simulink model "DC_motor_MPC"  (R2023a)
settings: Solver=FixedStepAuto  StartTime=0.0  StopTime=inf  FixedStep=0.002  RelTol=1e-3  EnableMultiTasking=on
values from neighbouring files (symbols this model uses):
  Npred = 20    [MPC_CasADi_2.m]
  Ts = 0.02    [MPC_CasADi_2.m]
undefined symbols (not defined in the file or in its folder): HIL, qc_get_step_size
libraries: quarc_library x33, dspbuff3 x12, simulink x7
settings Model: Creator=bajdus  LastModifiedBy=marinst
settings SolverCC: PositivePriorityOrder=on  AutoInsertRateTranBlk=on
settings RTWCC: Description=QUARC Win64 Target Using Toolchain  SystemTargetFile=quarc_win64.tlc  Toolchain=QUARC win64 | nmake (64-bit Windows)  BuildConfiguration=Faster Runs
settings STFCustomTargetCC: SystemTargetFile=quarc_win64.tlc
settings GRTTargetCC: ParMdlRefBuildCompliant=off  CompOptLevelCompliant=off  CombineOutputUpdateFcns=off  MatFileLogging=off  CPPClassGenCompliant=off  GRTInterface=on  ExtMode=on  ExtModeMexFile=quarc_comm

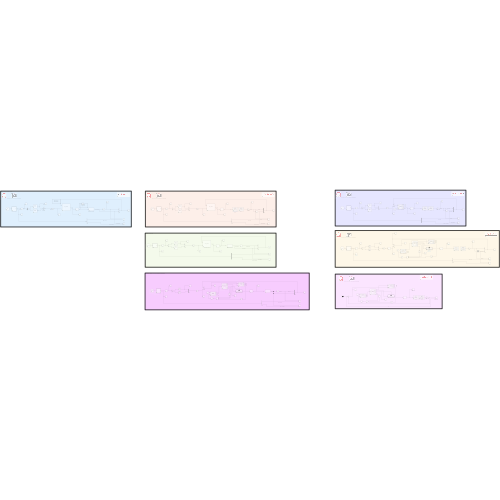
[thumbnail: Simulink's stored preview of the top-level diagram]
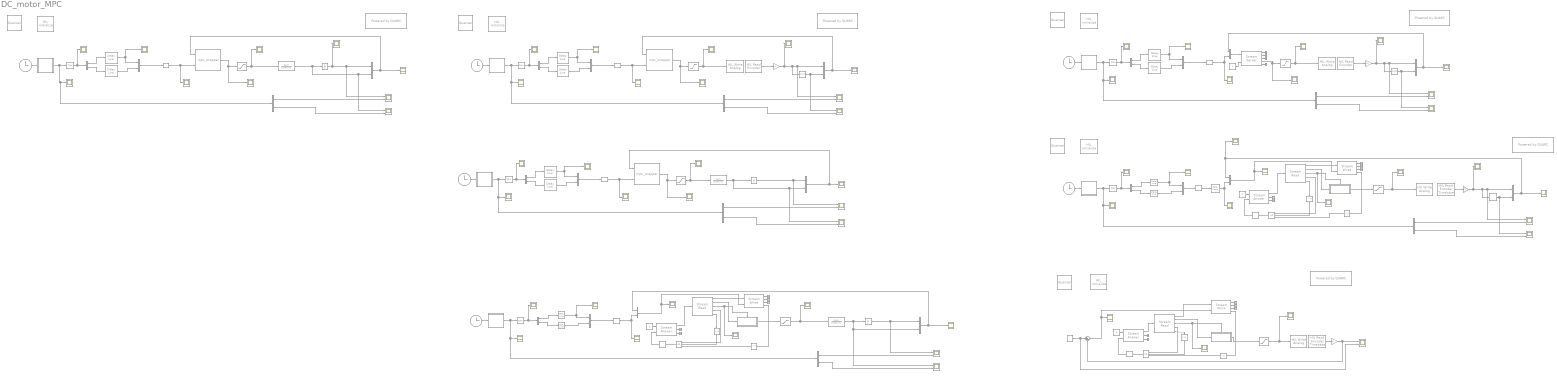
== system DC_motor_MPC ==
  note: QUARC Model PID - Server. Intermediate Communication
  note: Transfer function model
  note: QUARC Model
  note: QUARC Mode - Server. Basic Communication
  note: QUARC Model - Server. Intermediate Communication
  note: Mathematical Model - Server. Intermediate Communication
  note: QUARC Model - Transfer Function
  CasADi S-Function : S-Function  Commented=on  FunctionName=mpc_wrapper  SFunctionDeploymentMode=off  EnableBusSupport=off
  CasADi S-Function1 : S-Function  Commented=on  FunctionName=mpc_wrapper  SFunctionDeploymentMode=off  EnableBusSupport=off
  CasADi S-Function2 : S-Function  Commented=on  FunctionName=mpc_wrapper  SFunctionDeploymentMode=off  EnableBusSupport=off
  Clock{,1..5} (6 alike) : Clock  Commented=on
  Compare To Zero{,1..5} (6 alike) : simulink/Logic and Bit Operations/Compare To Zero  Commented=on  relop=<  OutDataTypeStr=boolean
  Constant : Constant  Commented=on
  Constant1 : Constant  Commented=on  Value=0
  Constant2 : Constant  Commented=on  Value=0
  Constant3 : Constant  Commented=on  Value=0
  Delay Line{,1..11} (12 alike) : dspbuff3/Delay Line  Commented=on  siz=Npred+1  ic=0  directfeed=off  enable_output=off  hold_output=off  OutputFrames=off
  Demux{,1..11} (12 alike) : Demux  Commented=on  Outputs=2
  Derivative : Derivative  Commented=on
  Derivative1 : Derivative  Commented=on
  Discrete Derivative : simulink/Discrete/Discrete Derivative  Commented=on  gainval=1.0  ICPrevScaledInput=0.0  OutMin=[]  OutMax=[]  OutDataType=fixdt(1, 16)  OutScaling=2^-10  DoSatur=off
  Enabled Subsystem : Subsystem  Commented=on  TreatAsAtomicUnit=on
  Enabled Subsystem1 : Subsystem  Commented=on  TreatAsAtomicUnit=on
  Enabled Subsystem2 : Subsystem  Commented=on  TreatAsAtomicUnit=on
  HIL Initialize : quarc_library/Data Acquisition/Generic/Configuration/HIL Initialize  Priority=-99  Commented=on  object_name=HIL-1  board_type=qube_servo3_usb  board_number=0@tcpip://localhost:18922  board_options=deadband_compensation=0.3;pwm_en=0;enc0_velocity=3.0;enc1_velocity=3.0;min_diode_compensation=0.3;max_diode_compensation=1.5  exclusive=off  active=off  hardware_clocks=[0]  clock_modes=[]  initial_clock_frequencies=[]  set_clock_params_at_start=off  set_clock_params_at_switch_in=off  set_clock_frequencies_at_start=off  set_clock_frequencies_at_switch_in=off  analog_input_channels=[0]  analog_input_configurations=[]  analog_input_maximums=3  analog_input_minimums=-3  set_analog_input_params_at_start=off  set_analog_input_params_at_switch_in=off  analog_output_channels=[0]  analog_output_maximums=15  analog_output_minimums=-15  initial_analog_outputs=[0]  final_analog_outputs=[0]  watchdog_analog_outputs=0  set_analog_output_params_at_start=off  set_analog_output_params_at_switch_in=off  set_analog_outputs_at_start=on  set_analog_outputs_at_switch_in=off  set_analog_outputs_at_terminate=on  set_analog_outputs_at_switch_out=off  set_analog_outputs_on_watchdog=on  digital_input_channels=[]  digital_output_channels=[0]  digital_output_configuration=[]  initial_digital_outputs=[1]  final_digital_outputs=[0]  watchdog_digital_outputs=[0]  set_digital_output_params_at_start=off  set_digital_output_params_at_switch_in=off  set_digital_outputs_at_start=on  set_digital_outputs_at_switch_in=off  set_digital_outputs_at_terminate=on  set_digital_outputs_at_switch_out=off  set_digital_outputs_on_watchdog=on  encoder_channels=[0:1]  quadrature=[4]  encoder_filter_frequency=[]  initial_encoder_counts=[0]  set_encoder_params_at_start=off  set_encoder_params_at_switch_in=off  set_encoder_counts_at_start=on  set_encoder_counts_at_switch_in=off  pwm_channels=[]  pwm_modes=[0]  pwm_frequency=23195  pwm_configuration=[1]  pwm_alignment=[0]  pwm_polarity=[1]  pwm_leading_deadband=[0]  pwm_trailing_deadband=[0]  initial_pwm_outputs=[0]  final_pwm_outputs=[0]  watchdog_pwm_outputs=[]  set_pwm_params_at_start=off  set_pwm_params_at_switch_in=off  set_pwm_outputs_at_start=off  set_pwm_outputs_at_switch_in=off  set_pwm_outputs_at_terminate=off  set_pwm_outputs_at_switch_out=off  set_pwm_outputs_on_watchdog=off  other_output_channels=[11000:11002]  initial_other_outputs=[0 1 0]  final_other_outputs=[1 0 0]  watchdog_other_outputs=[0 0 1]  set_other_outputs_at_start=on  set_other_outputs_at_switch_in=off  set_other_outputs_at_terminate=on  set_other_outputs_at_switch_out=off  set_other_outputs_on_watchdog=on
  HIL Initialize1 : quarc_library/Data Acquisition/Generic/Configuration/HIL Initialize  Priority=-99  Commented=on  object_name=HIL-1  board_type=qube_servo3_usb  board_number=0@tcpip://localhost:18922  board_options=deadband_compensation=0.3;pwm_en=0;enc0_velocity=3.0;enc1_velocity=3.0;min_diode_compensation=0.3;max_diode_compensation=1.5  exclusive=off  active=off  hardware_clocks=[0]  clock_modes=[]  initial_clock_frequencies=[]  set_clock_params_at_start=off  set_clock_params_at_switch_in=off  set_clock_frequencies_at_start=off  set_clock_frequencies_at_switch_in=off  analog_input_channels=[0]  analog_input_configurations=[]  analog_input_maximums=3  analog_input_minimums=-3  set_analog_input_params_at_start=off  set_analog_input_params_at_switch_in=off  analog_output_channels=[0]  analog_output_maximums=15  analog_output_minimums=-15  initial_analog_outputs=[0]  final_analog_outputs=[0]  watchdog_analog_outputs=0  set_analog_output_params_at_start=off  set_analog_output_params_at_switch_in=off  set_analog_outputs_at_start=on  set_analog_outputs_at_switch_in=off  set_analog_outputs_at_terminate=on  set_analog_outputs_at_switch_out=off  set_analog_outputs_on_watchdog=on  digital_input_channels=[]  digital_output_channels=[0]  digital_output_configuration=[]  initial_digital_outputs=[1]  final_digital_outputs=[0]  watchdog_digital_outputs=[0]  set_digital_output_params_at_start=off  set_digital_output_params_at_switch_in=off  set_digital_outputs_at_start=on  set_digital_outputs_at_switch_in=off  set_digital_outputs_at_terminate=on  set_digital_outputs_at_switch_out=off  set_digital_outputs_on_watchdog=on  encoder_channels=[0:1]  quadrature=[4]  encoder_filter_frequency=[]  initial_encoder_counts=[0]  set_encoder_params_at_start=off  set_encoder_params_at_switch_in=off  set_encoder_counts_at_start=on  set_encoder_counts_at_switch_in=off  pwm_channels=[]  pwm_modes=[0]  pwm_frequency=23195  pwm_configuration=[1]  pwm_alignment=[0]  pwm_polarity=[1]  pwm_leading_deadband=[0]  pwm_trailing_deadband=[0]  initial_pwm_outputs=[0]  final_pwm_outputs=[0]  watchdog_pwm_outputs=[]  set_pwm_params_at_start=off  set_pwm_params_at_switch_in=off  set_pwm_outputs_at_start=off  set_pwm_outputs_at_switch_in=off  set_pwm_outputs_at_terminate=off  set_pwm_outputs_at_switch_out=off  set_pwm_outputs_on_watchdog=off  other_output_channels=[11000:11002]  initial_other_outputs=[0 1 0]  final_other_outputs=[1 0 0]  watchdog_other_outputs=[0 0 1]  set_other_outputs_at_start=on  set_other_outputs_at_switch_in=off  set_other_outputs_at_terminate=on  set_other_outputs_at_switch_out=off  set_other_outputs_on_watchdog=on
  HIL Initialize2 : quarc_library/Data Acquisition/Generic/Configuration/HIL Initialize  Priority=-99  Commented=on  object_name=HIL-2  board_type=qube_servo3_usb  board_number=0@tcpip://localhost:18922  board_options=deadband_compensation=0.3;pwm_en=0;enc0_velocity=3.0;enc1_velocity=3.0;min_diode_compensation=0.3;max_diode_compensation=1.5  exclusive=off  active=off  hardware_clocks=[0]  clock_modes=[]  initial_clock_frequencies=[]  set_clock_params_at_start=off  set_clock_params_at_switch_in=off  set_clock_frequencies_at_start=off  set_clock_frequencies_at_switch_in=off  analog_input_channels=[0]  analog_input_configurations=[]  analog_input_maximums=3  analog_input_minimums=-3  set_analog_input_params_at_start=off  set_analog_input_params_at_switch_in=off  analog_output_channels=[0]  analog_output_maximums=15  analog_output_minimums=-15  initial_analog_outputs=[0]  final_analog_outputs=[0]  watchdog_analog_outputs=0  set_analog_output_params_at_start=off  set_analog_output_params_at_switch_in=off  set_analog_outputs_at_start=on  set_analog_outputs_at_switch_in=off  set_analog_outputs_at_terminate=on  set_analog_outputs_at_switch_out=off  set_analog_outputs_on_watchdog=on  digital_input_channels=[]  digital_output_channels=[0]  digital_output_configuration=[]  initial_digital_outputs=[1]  final_digital_outputs=[0]  watchdog_digital_outputs=[0]  set_digital_output_params_at_start=off  set_digital_output_params_at_switch_in=off  set_digital_outputs_at_start=on  set_digital_outputs_at_switch_in=off  set_digital_outputs_at_terminate=on  set_digital_outputs_at_switch_out=off  set_digital_outputs_on_watchdog=on  encoder_channels=[0:1]  quadrature=[4]  encoder_filter_frequency=[]  initial_encoder_counts=[0]  set_encoder_params_at_start=off  set_encoder_params_at_switch_in=off  set_encoder_counts_at_start=on  set_encoder_counts_at_switch_in=off  pwm_channels=[]  pwm_modes=[0]  pwm_frequency=23195  pwm_configuration=[1]  pwm_alignment=[0]  pwm_polarity=[1]  pwm_leading_deadband=[0]  pwm_trailing_deadband=[0]  initial_pwm_outputs=[0]  final_pwm_outputs=[0]  watchdog_pwm_outputs=[]  set_pwm_params_at_start=off  set_pwm_params_at_switch_in=off  set_pwm_outputs_at_start=off  set_pwm_outputs_at_switch_in=off  set_pwm_outputs_at_terminate=off  set_pwm_outputs_at_switch_out=off  set_pwm_outputs_on_watchdog=off  other_output_channels=[11000:11002]  initial_other_outputs=[0 1 0]  final_other_outputs=[1 0 0]  watchdog_other_outputs=[0 0 1]  set_other_outputs_at_start=on  set_other_outputs_at_switch_in=off  set_other_outputs_at_terminate=on  set_other_outputs_at_switch_out=off  set_other_outputs_on_watchdog=on
  HIL Initialize3 : quarc_library/Data Acquisition/Generic/Configuration/HIL Initialize  Priority=-99  Commented=on  object_name=HIL-1  board_type=qube_servo3_usb  board_number=0@tcpip://localhost:18922  board_options=deadband_compensation=0.3;pwm_en=0;enc0_velocity=3.0;enc1_velocity=3.0;min_diode_compensation=0.3;max_diode_compensation=1.5  exclusive=off  active=off  hardware_clocks=[0]  clock_modes=[]  initial_clock_frequencies=[]  set_clock_params_at_start=off  set_clock_params_at_switch_in=off  set_clock_frequencies_at_start=off  set_clock_frequencies_at_switch_in=off  analog_input_channels=[0]  analog_input_configurations=[]  analog_input_maximums=3  analog_input_minimums=-3  set_analog_input_params_at_start=off  set_analog_input_params_at_switch_in=off  analog_output_channels=[0]  analog_output_maximums=15  analog_output_minimums=-15  initial_analog_outputs=[0]  final_analog_outputs=[0]  watchdog_analog_outputs=0  set_analog_output_params_at_start=off  set_analog_output_params_at_switch_in=off  set_analog_outputs_at_start=on  set_analog_outputs_at_switch_in=off  set_analog_outputs_at_terminate=on  set_analog_outputs_at_switch_out=off  set_analog_outputs_on_watchdog=on  digital_input_channels=[]  digital_output_channels=[0]  digital_output_configuration=[]  initial_digital_outputs=[1]  final_digital_outputs=[0]  watchdog_digital_outputs=[0]  set_digital_output_params_at_start=off  set_digital_output_params_at_switch_in=off  set_digital_outputs_at_start=on  set_digital_outputs_at_switch_in=off  set_digital_outputs_at_terminate=on  set_digital_outputs_at_switch_out=off  set_digital_outputs_on_watchdog=on  encoder_channels=[0:1]  quadrature=[4]  encoder_filter_frequency=[]  initial_encoder_counts=[0]  set_encoder_params_at_start=off  set_encoder_params_at_switch_in=off  set_encoder_counts_at_start=on  set_encoder_counts_at_switch_in=off  pwm_channels=[]  pwm_modes=[0]  pwm_frequency=23195  pwm_configuration=[1]  pwm_alignment=[0]  pwm_polarity=[1]  pwm_leading_deadband=[0]  pwm_trailing_deadband=[0]  initial_pwm_outputs=[0]  final_pwm_outputs=[0]  watchdog_pwm_outputs=[]  set_pwm_params_at_start=off  set_pwm_params_at_switch_in=off  set_pwm_outputs_at_start=off  set_pwm_outputs_at_switch_in=off  set_pwm_outputs_at_terminate=off  set_pwm_outputs_at_switch_out=off  set_pwm_outputs_on_watchdog=off  other_output_channels=[11000:11002]  initial_other_outputs=[0 1 0]  final_other_outputs=[1 0 0]  watchdog_other_outputs=[0 0 1]  set_other_outputs_at_start=on  set_other_outputs_at_switch_in=off  set_other_outputs_at_terminate=on  set_other_outputs_at_switch_out=off  set_other_outputs_on_watchdog=on
  HIL Initialize4 : quarc_library/Data Acquisition/Generic/Configuration/HIL Initialize  Priority=-99  Commented=on  object_name=HIL-2  board_type=qube_servo3_usb  board_number=0@tcpip://localhost:18922  board_options=deadband_compensation=0.3;pwm_en=0;enc0_velocity=3.0;enc1_velocity=3.0;min_diode_compensation=0.3;max_diode_compensation=1.5  exclusive=off  active=off  hardware_clocks=[0]  clock_modes=[]  initial_clock_frequencies=[]  set_clock_params_at_start=off  set_clock_params_at_switch_in=off  set_clock_frequencies_at_start=off  set_clock_frequencies_at_switch_in=off  analog_input_channels=[0]  analog_input_configurations=[]  analog_input_maximums=3  analog_input_minimums=-3  set_analog_input_params_at_start=off  set_analog_input_params_at_switch_in=off  analog_output_channels=[0]  analog_output_maximums=15  analog_output_minimums=-15  initial_analog_outputs=[0]  final_analog_outputs=[0]  watchdog_analog_outputs=0  set_analog_output_params_at_start=off  set_analog_output_params_at_switch_in=off  set_analog_outputs_at_start=on  set_analog_outputs_at_switch_in=off  set_analog_outputs_at_terminate=on  set_analog_outputs_at_switch_out=off  set_analog_outputs_on_watchdog=on  digital_input_channels=[]  digital_output_channels=[0]  digital_output_configuration=[]  initial_digital_outputs=[1]  final_digital_outputs=[0]  watchdog_digital_outputs=[0]  set_digital_output_params_at_start=off  set_digital_output_params_at_switch_in=off  set_digital_outputs_at_start=on  set_digital_outputs_at_switch_in=off  set_digital_outputs_at_terminate=on  set_digital_outputs_at_switch_out=off  set_digital_outputs_on_watchdog=on  encoder_channels=[0:1]  quadrature=[4]  encoder_filter_frequency=[]  initial_encoder_counts=[0]  set_encoder_params_at_start=off  set_encoder_params_at_switch_in=off  set_encoder_counts_at_start=on  set_encoder_counts_at_switch_in=off  pwm_channels=[]  pwm_modes=[0]  pwm_frequency=23195  pwm_configuration=[1]  pwm_alignment=[0]  pwm_polarity=[1]  pwm_leading_deadband=[0]  pwm_trailing_deadband=[0]  initial_pwm_outputs=[0]  final_pwm_outputs=[0]  watchdog_pwm_outputs=[]  set_pwm_params_at_start=off  set_pwm_params_at_switch_in=off  set_pwm_outputs_at_start=off  set_pwm_outputs_at_switch_in=off  set_pwm_outputs_at_terminate=off  set_pwm_outputs_at_switch_out=off  set_pwm_outputs_on_watchdog=off  other_output_channels=[11000:11002]  initial_other_outputs=[0 1 0]  final_other_outputs=[1 0 0]  watchdog_other_outputs=[0 0 1]  set_other_outputs_at_start=on  set_other_outputs_at_switch_in=off  set_other_outputs_at_terminate=on  set_other_outputs_at_switch_out=off  set_other_outputs_on_watchdog=on
  HIL Read Encoder : quarc_library/Data Acquisition/Generic/Immediate I//O/HIL Read Encoder  Commented=on  object_name=HIL-1  channels=0  sample_time=qc_get_step_size  active=on  vector_output=off  data_type_mode=Inherit via back propagation  data_type=double
  HIL Read Encoder Timebase : quarc_library/Data Acquisition/Generic/Timebases/HIL Read Encoder Timebase  Commented=on  object_name=HIL-2  clock=0  channels=0  active=on  vector_output=off  data_type_mode=Inherit via back propagation  data_type=double  overflow_mode=Error on overflow  samples_in_buffer=max(ceil(1/qc_get_step_size), 1)
  HIL Read Encoder Timebase1 : quarc_library/Data Acquisition/Generic/Timebases/HIL Read Encoder Timebase  Commented=on  object_name=HIL-1  clock=0  channels=0  active=on  vector_output=off  data_type_mode=Inherit via back propagation  data_type=double  overflow_mode=Error on overflow  samples_in_buffer=max(ceil(1/qc_get_step_size), 1)
  HIL Read Encoder1 : quarc_library/Data Acquisition/Generic/Immediate I//O/HIL Read Encoder  Commented=on  object_name=HIL-1  channels=0  sample_time=qc_get_step_size  active=on  vector_output=off  data_type_mode=Inherit via back propagation  data_type=double
  HIL Write Analog : quarc_library/Data Acquisition/Generic/Immediate I//O/HIL Write Analog  Commented=on  object_name=HIL-1  channels=0  sample_time=-1  active=off  vector_input=off
  HIL Write Analog1 : quarc_library/Data Acquisition/Generic/Immediate I//O/HIL Write Analog  Commented=on  object_name=HIL-1  channels=0  sample_time=-1  active=off  vector_input=off
  HIL Write Analog2 : quarc_library/Data Acquisition/Generic/Immediate I//O/HIL Write Analog  Commented=on  object_name=HIL-2  channels=0  sample_time=-1  active=off  vector_input=off
  HIL Write Analog3 : quarc_library/Data Acquisition/Generic/Immediate I//O/HIL Write Analog  Commented=on  object_name=HIL-1  channels=0  sample_time=-1  active=off  vector_input=off
  Integrator : Integrator  Commented=on
  Integrator1 : Integrator  Commented=on
  Integrator2 : Integrator  Commented=on
  Logical Operator : Logic  Commented=on  Operator=OR  Inputs=3  AllPortsSameDT=off  OutDataTypeStr=boolean
  Logical Operator1 : Logic  Commented=on  Operator=OR  Inputs=3  AllPortsSameDT=off  OutDataTypeStr=boolean
  Logical Operator2 : Logic  Commented=on  Operator=OR  Inputs=3  AllPortsSameDT=off  OutDataTypeStr=boolean
  MATLAB Function : MATLAB Function  Commented=on  TreatAsAtomicUnit=on
  MATLAB Function1 : MATLAB Function  Commented=on  TreatAsAtomicUnit=on
  MATLAB Function2 : MATLAB Function  Commented=on  TreatAsAtomicUnit=on
  MATLAB Function3 : MATLAB Function  Commented=on  TreatAsAtomicUnit=on
  MATLAB Function4 : MATLAB Function  Commented=on  TreatAsAtomicUnit=on
  MATLAB Function5 : MATLAB Function  Commented=on  TreatAsAtomicUnit=on
  Memory : Memory  Commented=on
  Memory1 : Memory  Commented=on
  Memory2 : Memory  Commented=on
  Mux{,1..5,7..8,10..11,13..14} (12 alike) : Mux  Commented=on  Inputs=2
  Mux12 : Mux  Commented=on  Inputs=[2 42]
  Mux6 : Mux  Commented=on  Inputs=[2 42]
  Mux9 : Mux  Commented=on  Inputs=[2 42]
  Position (rad) : Scope  Commented=on  NumInputPorts=2
  Powered by QUARC{,1..4} (5 alike) : quarc_library/Logos/Powered by QUARC  Commented=on
  QUBE-Servo Model1 : TransferFcn  Commented=on  Numerator=[26.5]  Denominator=[0.097 1]
  QUBE-Servo Model2 : TransferFcn  Commented=on  Numerator=[26.5]  Denominator=[0.097 1]
  QUBE-Servo Model3 : TransferFcn  Commented=on  Numerator=[26.5]  Denominator=[0.097 1]
  Quanser{,1..4} (5 alike) : quarc_library/Logos/Quanser  Commented=on
  Rate Transition : RateTransition  Commented=on
  Reshape{,1..5} (6 alike) : Reshape  Commented=on
  Saturation{,1..6} (7 alike) : Saturate  Commented=on  UpperLimit=10  LowerLimit=-10
  Scope{,1..2,4..10,12..13,15..17,19..20,23..30,33..41,44..54,57..62} (51 alike) : Scope  Commented=on
  Scope{3,11,14,18,21..22,31..32,42..43,55..56} (12 alike) : Scope  Commented=on  NumInputPorts=2
  Square Wave Generator : SignalGenerator  Commented=on  WaveForm=square  Amplitude=pi/4  Frequency=0.5
  Stream Answer : quarc_library/Communications/Intermediate/Stream Answer  Commented=on  uri_source=Specify via dialog (do not evaluate)  uri=tcpip://localhost:18001  send_buffer_size=8000  receive_buffer_size=8000  byte_order=little endian (Intel - LSB first)  sample_time=qc_get_step_size  active=on
      settings: AttributesFormatString="\"tcpip://localhost:18001\""  SourceProductName=QUARC Targets
  Stream Answer1 : quarc_library/Communications/Intermediate/Stream Answer  Commented=on  uri_source=Specify via dialog (do not evaluate)  uri=tcpip://localhost:18001  send_buffer_size=8000  receive_buffer_size=8000  byte_order=little endian (Intel - LSB first)  sample_time=qc_get_step_size  active=on
      settings: AttributesFormatString="\"tcpip://localhost:18001\""  SourceProductName=QUARC Targets
  Stream Answer2 : quarc_library/Communications/Intermediate/Stream Answer  Commented=on  uri_source=Specify via dialog (do not evaluate)  uri=tcpip://localhost:18001  send_buffer_size=8000  receive_buffer_size=8000  byte_order=little endian (Intel - LSB first)  sample_time=qc_get_step_size  active=on
      settings: AttributesFormatString="\"tcpip://localhost:18001\""  SourceProductName=QUARC Targets
  Stream Read : quarc_library/Communications/Intermediate/Stream Read  Commented=on  data_type=double  type_expr=BusObject  num_elements=1  receive_dims=off
      settings: SourceProductName=QUARC Targets
  Stream Read1 : quarc_library/Communications/Intermediate/Stream Read  Commented=on  data_type=double  type_expr=BusObject  num_elements=1  receive_dims=off
      settings: SourceProductName=QUARC Targets
  Stream Read2 : quarc_library/Communications/Intermediate/Stream Read  Commented=on  data_type=double  type_expr=BusObject  num_elements=1  receive_dims=off
      settings: SourceProductName=QUARC Targets
  Stream Server : quarc_library/Communications/Basic/Stream Server  Commented=on  uri_source=Specify via dialog (do not evaluate)  uri=tcpip://localhost:18001  send_buffer_size=1460  receive_buffer_size=1460  byte_order=little endian (Intel - LSB first)  optimization=Minimum latency  send_options=Send all data  receive_options=Receive all data  default_value=[0]  sample_time=qc_get_step_size  active=off  implementation=Use blocking I/O in a separate thread  send_fifo_size=1000  receive_fifo_size=1000  send_priority=0  receive_priority=0  send_dimensions=off  receive_dimensions=off  max_dimensions=-1  data_type=Inherited via back propagation  type_expr=BusObject
      settings: AttributesFormatString="\"tcpip://localhost:18001\""
  Stream Write : quarc_library/Communications/Intermediate/Stream Write  Commented=on  optimization=Minimizing latency  send_dims=off
      settings: SourceProductName=QUARC Targets
  Stream Write1 : quarc_library/Communications/Intermediate/Stream Write  Commented=on  optimization=Minimizing latency  send_dims=off
      settings: SourceProductName=QUARC Targets
  Stream Write2 : quarc_library/Communications/Intermediate/Stream Write  Commented=on  optimization=Minimizing latency  send_dims=off
      settings: SourceProductName=QUARC Targets
  Sum1 : Sum  Commented=on  Inputs=|+-
  Terminator{,1..18} (19 alike) : Terminator  Commented=on
  Voltage (V)1 : Scope  Commented=on
  Zero-Order Hold{,1..5} (6 alike) : ZeroOrderHold  Commented=on  SampleTime=Ts
  counts to rad{,1..3} (4 alike) : Gain  Commented=on  Gain=2*pi/512/4
  wires:
  Saturation/1 -> HIL Write Analog/1, Scope5/1  "u(V)"
  CasADi S-Function/1 -> Scope1/1, Saturation/1  "u (V)"
  counts to rad/1 -> Scope3/1, Mux2/1, Derivative/1, Scope6/1  "theta (rad)"
  Derivative/1 -> Scope18/1, Mux2/2  "omega (rad/sec)"
  Mux2/1 -> Scope/1, CasADi S-Function/1
  Clock/1 -> MATLAB Function/1(t)
  MATLAB Function/1(ref) -> Demux3/1, Scope4/1, Zero-Order Hold/1  "x_ref"
  Mux/1 -> Reshape/1
  Zero-Order Hold/1 -> Demux/1, Scope7/1
  Reshape/1 -> Scope8/1, CasADi S-Function/2  "xref"
  Demux/1 -> Delay Line/1
  Demux/2 -> Delay Line1/1
  Delay Line/1 -> Mux/1, Scope9/1
  Delay Line1/1 -> Mux/2
  HIL Read Encoder/1 -> counts to rad/1
  QUBE-Servo Model2/1 -> Scope11/1, Mux3/2, Integrator/1  "speed(rad/sec)"
  Delay Line3/1 -> Mux1/2
  Demux1/2 -> Delay Line3/1
  Saturation1/1 -> QUBE-Servo Model2/1, Scope13/1  "u(V)"
  Delay Line2/1 -> Mux1/1, Scope17/1
  Demux1/1 -> Delay Line2/1
  Zero-Order Hold1/1 -> Demux1/1, Scope15/1
  MATLAB Function1/1(ref) -> Demux2/1, Scope12/1, Zero-Order Hold1/1  "x_ref"
  Clock1/1 -> MATLAB Function1/1(t)
  Mux1/1 -> Reshape1/1
  Mux3/1 -> CasADi S-Function1/1, Scope2/1
  CasADi S-Function1/1 -> Scope10/1, Saturation1/1  "u (V)"
  Integrator/1 -> Scope14/1, Mux3/1  "position (rad/sec)"
  Reshape1/1 -> Scope16/1, CasADi S-Function1/2  "xref"
  Demux2/1 -> Scope14/2  "theta_ref (rad)"
  Demux2/2 -> Scope11/2  "omega_ref (rad/sec)"
  Demux3/2 -> Scope18/2  "omega_ref (rad/sec)"
  Demux3/1 -> Scope3/2  "theta_ref (rad)"
  Demux5/1 -> Scope22/2  "theta_ref (rad)"
  Saturation2/1 -> HIL Write Analog1/1, Scope24/1  "u(V)"
  HIL Read Encoder1/1 -> counts to rad1/1
  MATLAB Function2/1(ref) -> Demux5/1, Scope23/1, Zero-Order Hold2/1  "x_ref"
  Clock2/1 -> MATLAB Function2/1(t)
  Derivative1/1 -> Scope21/1, Mux5/2  "omega (rad/sec)"
  Demux4/2 -> Delay Line5/1
  Demux4/1 -> Delay Line4/1
  Delay Line5/1 -> Mux4/2
  Mux4/1 -> Reshape2/1
  Stream Server/4 -> Scope20/1, Saturation2/1  "u (V)"
  Reshape2/1 -> Mux6/2, Scope27/1  "xref"
  Demux5/2 -> Scope21/2  "omega_ref (rad/sec)"
  Mux5/1 -> Mux6/1, Scope19/1  "x0"
  counts to rad1/1 -> Scope22/1, Mux5/1, Derivative1/1, Scope25/1  "theta (rad)"
  Delay Line4/1 -> Mux4/1, Scope28/1
  Zero-Order Hold2/1 -> Demux4/1, Scope26/1
  Mux6/1 -> Stream Server/1
  Constant/1 -> Stream Server/2
  Stream Server/1 -> Terminator/1
  Stream Server/2 -> Terminator1/1
  Stream Server/3 -> Terminator2/1
  Stream Server/5 -> Terminator3/1
  Stream Answer/3 -> Terminator7/1
  Stream Write/4 -> Compare To Zero1/1
  Constant1/1 -> Stream Answer/1
  Stream Read/5 -> Compare To Zero/1
  Stream Read/4 -> Logical Operator/1
  Logical Operator/1 -> Memory/1
  Stream Write/1 -> Terminator5/1
  Stream Answer/1 -> Stream Read/1
  Stream Read/3 -> Enabled Subsystem1/Enable, Scope39/1
  Stream Answer/2 -> Terminator6/1
  Memory/1 -> Stream Answer/2
  Stream Read/1 -> Stream Write/1
  Stream Write/2 -> Terminator8/1
  Stream Write/3 -> Terminator9/1
  Reshape3/1 -> Rate Transition/1  "xref"
  Saturation3/1 -> HIL Write Analog2/1, Scope34/1  "u(V)"
  Mux7/1 -> Reshape3/1
  counts to rad2/1 -> Discrete Derivative/1, Scope32/1, Mux8/1, Scope35/1  "theta (rad)"
  Delay Line6/1 -> Scope38/1, Mux7/1
  Zero-Order Hold3/1 -> Demux6/1, Scope36/1
  Demux7/2 -> Scope31/2  "omega_ref (rad/sec)"
  Mux8/1 -> Mux9/1, Scope46/1, Scope29/1  "x0"
  Discrete Derivative/1 -> Scope31/1, Mux8/2  "omega (rad/sec)"
  Demux6/1 -> Delay Line6/1
  Delay Line7/1 -> Mux7/2
  Demux6/2 -> Delay Line7/1
  Demux7/1 -> Scope32/2  "theta_ref (rad)"
  MATLAB Function3/1(ref) -> Demux7/1, Scope33/1, Zero-Order Hold3/1  "x_ref"
  Mux9/1 -> Scope30/1, Stream Write/2
  HIL Read Encoder Timebase/1 -> counts to rad2/1
  Clock3/1 -> MATLAB Function3/1(t)
  Stream Read/2 -> Enabled Subsystem1/1(In1)
  Enabled Subsystem1/1(Out1) -> Saturation3/1
  Compare To Zero/1 -> Logical Operator/2
  Compare To Zero1/1 -> Logical Operator/3
  Stream Read1/3 -> Enabled Subsystem2/Enable, Scope50/1
  Integrator1/1 -> Scope43/1, Mux11/1  "theta (rad)"
  Saturation4/1 -> QUBE-Servo Model1/1, Scope45/1  "u(V)"
  Clock4/1 -> MATLAB Function4/1(t)
  MATLAB Function4/1(ref) -> Demux9/1, Scope44/1, Zero-Order Hold4/1  "x_ref"
  Stream Answer1/2 -> Terminator10/1
  Stream Answer1/3 -> Terminator11/1
  Mux10/1 -> Reshape4/1
  Demux8/1 -> Delay Line8/1
  Compare To Zero2/1 -> Logical Operator1/2
  Stream Write1/3 -> Terminator13/1
  Delay Line8/1 -> Scope49/1, Mux10/1
  Stream Read1/4 -> Logical Operator1/1
  Reshape4/1 -> Mux12/2, Scope48/1  "xref"
  Logical Operator1/1 -> Memory1/1
  Stream Read1/1 -> Stream Write1/1
  Stream Read1/5 -> Compare To Zero2/1
  Zero-Order Hold4/1 -> Demux8/1, Scope47/1
  Stream Write1/1 -> Terminator4/1
  Demux9/1 -> Scope43/2  "theta_ref (rad)"
  Demux9/2 -> Scope42/2  "omega_ref (rad/sec)"
  Compare To Zero3/1 -> Logical Operator1/3
  Demux8/2 -> Delay Line9/1
  Mux11/1 -> Mux12/1, Scope40/1  "x0"
  Delay Line9/1 -> Mux10/2
  Memory1/1 -> Stream Answer1/2
  Stream Write1/2 -> Terminator12/1
  Constant2/1 -> Stream Answer1/1
  Mux12/1 -> Scope41/1, Stream Write1/2
  Enabled Subsystem2/1(Out1) -> Saturation4/1
  Stream Write1/4 -> Compare To Zero3/1
  Stream Answer1/1 -> Stream Read1/1
  Stream Read1/2 -> Enabled Subsystem2/1(In1)
  QUBE-Servo Model1/1 -> Scope42/1, Mux11/2, Integrator1/1  "speed(rad/sec)"
  counts to rad3/1 -> Position (rad)/1, Sum1/2  "y"
  HIL Read Encoder Timebase1/1 -> counts to rad3/1
  Square Wave Generator/1 -> Sum1/1, Position (rad)/2  "ref"
  Saturation6/1 -> HIL Write Analog3/1, Voltage (V)1/1
  Stream Write2/3 -> Terminator18/1
  Stream Answer2/2 -> Terminator15/1
  Stream Read2/3 -> Enabled Subsystem/Enable, Scope52/1
  Compare To Zero4/1 -> Logical Operator2/2
  Memory2/1 -> Stream Answer2/2
  Sum1/1 -> Stream Write2/2, Scope51/1
  Stream Read2/2 -> Enabled Subsystem/1(In1)
  Stream Write2/2 -> Terminator17/1
  Enabled Subsystem/1(Out1) -> Saturation6/1
  Compare To Zero5/1 -> Logical Operator2/3
  Stream Answer2/3 -> Terminator16/1
  Stream Read2/4 -> Logical Operator2/1
  Stream Write2/4 -> Compare To Zero5/1
  Logical Operator2/1 -> Memory2/1
  Stream Read2/1 -> Stream Write2/1
  Stream Read2/5 -> Compare To Zero4/1
  Stream Answer2/1 -> Stream Read2/1
  Constant3/1 -> Stream Answer2/1
  Stream Write2/1 -> Terminator14/1
  Rate Transition/1 -> Mux9/2, Scope37/1
  Clock5/1 -> MATLAB Function5/1(t)
  QUBE-Servo Model3/1 -> Scope55/1, Mux14/2, Integrator2/1  "omega (rad/sec)"
  Mux14/1 -> Scope53/1, CasADi S-Function2/1
  Demux11/2 -> Scope55/2  "omega_ref (rad/sec)"
  CasADi S-Function2/1 -> Scope54/1, Saturation5/1  "u (V)"
  Saturation5/1 -> QUBE-Servo Model3/1, Scope58/1  "u(V)"
  Reshape5/1 -> Scope61/1, CasADi S-Function2/2  "xref"
  Zero-Order Hold5/1 -> Demux10/1, Scope60/1
  Demux10/1 -> Delay Line10/1
  Delay Line11/1 -> Mux13/2
  Mux13/1 -> Reshape5/1
  Demux11/1 -> Scope56/2  "theta_ref (rad)"
  Delay Line10/1 -> Mux13/1, Scope62/1
  Demux10/2 -> Delay Line11/1
  MATLAB Function5/1(ref) -> Demux11/1, Scope57/1, Zero-Order Hold5/1  "x_ref"
  Integrator2/1 -> Scope56/1, Mux14/1, Scope59/1

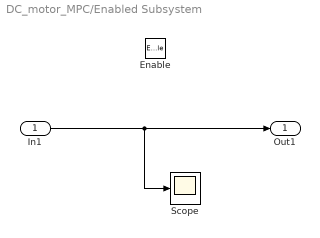
== system DC_motor_MPC/Enabled Subsystem ==
  In1 : Inport
  Enable : EnablePort
  Scope : Scope
  Out1 : Outport
  wires:
  In1/1 -> Scope/1, Out1/1

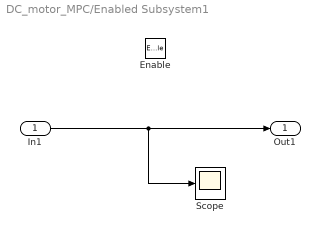
== system DC_motor_MPC/Enabled Subsystem1 ==
  In1 : Inport
  Enable : EnablePort
  Scope : Scope
  Out1 : Outport
  wires:
  In1/1 -> Scope/1, Out1/1

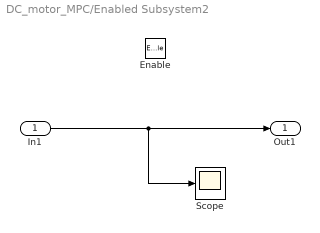
== system DC_motor_MPC/Enabled Subsystem2 ==
  In1 : Inport
  Enable : EnablePort
  Scope : Scope
  Out1 : Outport
  wires:
  In1/1 -> Scope/1, Out1/1

== matlab function DC_motor_MPC/MATLAB Function1 ==
  data: t input; ref output
function ref = generate_ref(t)
    amp = pi/4;
    freq = 0.5;
    ref1 = -amp * square(2*pi*freq*t);
    ref2 = 0;
    ref = [ref1; ref2];
end

== matlab function DC_motor_MPC/MATLAB Function ==
  data: t input; ref output
function ref = generate_ref(t)
    amp = pi/4;
    freq = 0.5;
    ref1 = -amp * square(2*pi*freq*t);
    ref2 = 0;
    ref = [ref1; ref2];
end

== matlab function DC_motor_MPC/MATLAB Function2 ==
  data: t input; ref output
function ref = generate_ref(t)
    amp = pi/4;
    freq = 0.5;
    ref1 = -amp * square(2*pi*freq*t);
    ref2 = 0;
    ref = [ref1; ref2];
end

== matlab function DC_motor_MPC/MATLAB Function3 ==
  data: t input; ref output
function ref = generate_ref(t)
    amp = pi/4;
    freq = 0.5;
    ref1 = -amp * square(2*pi*freq*t);
    ref2 = 0;
    ref = [ref1; ref2];
end

== matlab function DC_motor_MPC/MATLAB Function4 ==
  data: t input; ref output
function ref = generate_ref(t)
    amp = pi/4;
    freq = 0.5;
    ref1 = -amp * square(2*pi*freq*t);
    ref2 = 0;
    ref = [ref1; ref2];
end

== matlab function DC_motor_MPC/MATLAB Function5 ==
  data: t input; ref output
function ref = generate_ref(t)
    amp = pi/4;
    freq = 0.5;
    ref1 = -amp * square(2*pi*freq*t);
    ref2 = 0;
    ref = [ref1; ref2];
end
